simulink model "Inverter_Bipolar_motor"  (R2024a)
settings: Solver=VariableStepAuto  StartTime=0.0  StopTime=2  RelTol=1e-3
undefined symbols (not defined in the file): Capacitor, Start
libraries: spsIGBTDiodeLib x4, spsCurrentMeasurementLib x2, spsDCVoltageSourceLib x1, simulink x1, spsSinglePhaseAsynchronousMachineLib x1, spsVoltageMeasurementLib x1, sps_lib x1
settings Model: Creator=yashg  LastModifiedBy=yashg

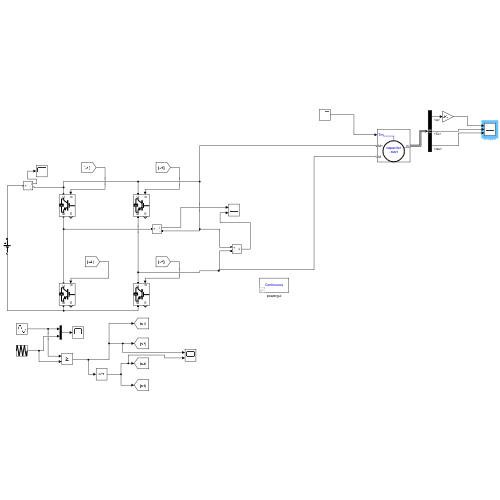
[thumbnail: Simulink's stored preview of the top-level diagram]
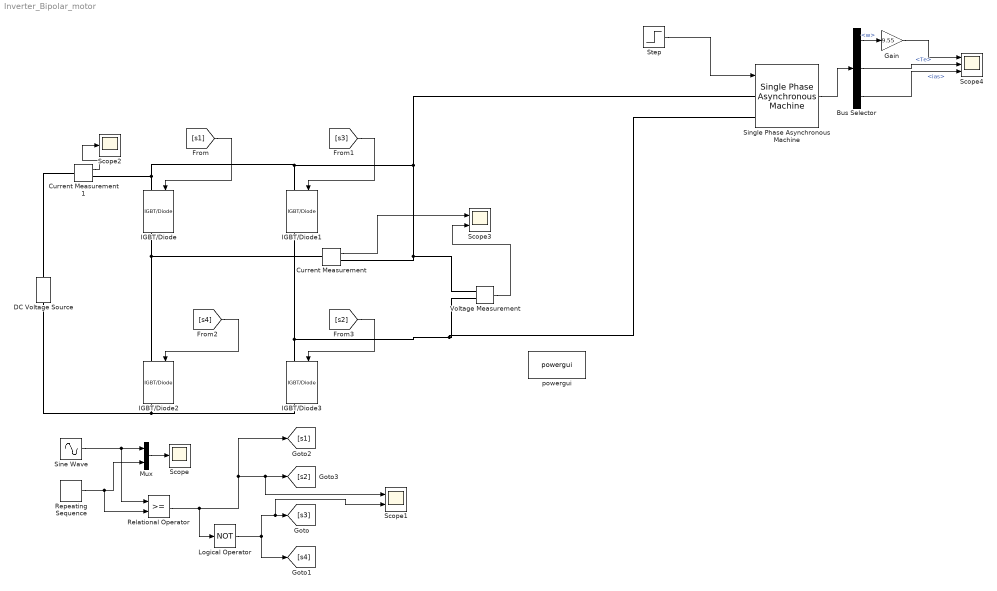
== system Inverter_Bipolar_motor ==
  Bus Selector : BusSelector  OutputSignals=w,Te,ias
  Current Measurement : spsCurrentMeasurementLib/Current Measurement  PhasorSimulation=off  OutputType=Complex  PSBequivalent=0
  Current Measurement1 : spsCurrentMeasurementLib/Current Measurement  PhasorSimulation=off  OutputType=Complex  PSBequivalent=0
  DC Voltage Source : spsDCVoltageSourceLib/DC Voltage Source  Amplitude=100  Measurements=None
  Gain : Gain  Gain=9.55
  IGBT/Diode{,1..3} (4 alike) : spsIGBTDiodeLib/IGBT//Diode  Ron=1e-3  Rs=1e5  Cs=inf  Measurements=on
  Logical Operator : Logic  Operator=NOT  AllPortsSameDT=off  OutDataTypeStr=boolean
  Mux : Mux  Inputs=2
  Relational Operator : RelationalOperator  OutDataTypeStr=boolean  RndMeth=Simplest  InputSameDT=off
  Repeating Sequence : simulink/Sources/Repeating Sequence  rep_seq_t=[0 1 2 3 4]*[1/400]  rep_seq_y=[0 1 0 -1 0]
  Scope : Scope
  Scope1 : Scope  NumInputPorts=2
  Scope2 : Scope
  Scope3 : Scope  NumInputPorts=2
  Scope4 : Scope  NumInputPorts=3
  Sine Wave : Sin  Frequency=2*pi*50  SampleTime=0
  Single Phase Asynchronous Machine : spsSinglePhaseAsynchronousMachineLib/Single Phase Asynchronous Machine  MechanicalLoad=Torque Tm  UNITS=SI  MachineType=Capacitor-Start  MeasurementBus=on  NominalParameters="[ .25*746  110  60]"  MainWindingStator="[2.02  7.4e-3]"  MainWindingRotor="[4.12  5.6e-3]"  MutualInductance=0.1772  AuxiliaryWinding="[7.14  8.5e-3]"  Mechanical="[0.0146  0  2 1.18]"  CapacitorStart="[2  254.7e-6]"  CapacitorRun="[18  21.1e-6]"  DisconnectionSpeed=75  InitialSpeed=0  DataType=SI  TsPowergui=0  TsBlock=-1
      settings: LibrarySourceBlock=|
      | sps_lib/Electrical Machines/Single Phase
      | Asynchronous Machine
  Step : Step  Time=0  After=10  SampleTime=0
  Voltage Measurement : spsVoltageMeasurementLib/Voltage Measurement  PhasorSimulation=off  OutputType=Complex  PSBequivalent=0
  powergui : sps_lib/powergui  Priority=1  SimulationMode=Continuous  SampleTime=50e-6  frequency=60  Iterations=50  frequencyindice=0  Pbase=100e6  ErrMax=1e-4  UnitsV=kV  UnitsW=MW  buscounter=0  FunctionMessages=off  echomessages=off  EnableUseOfTLC=off  CurrentSourceSwitches=off  DisableSnubberDevices=off  DisableRonSwitches=off  DisableVfSwitches=off  DisplayEquations=off  AutomaticDiscreteSolvers=off  SolverType=Tustin/Backward Euler (TBE)  Interpol=off  ExternalGateDelay=off  methode=off  Ts=100  x0status=blocks  SPID=on  SwTol=0  HookPort=off  NonlinearTolerance=1e-4  nMaxIteration=100  ContinueOnMaxIteration=off  RestoreLinks=warning  ResistiveCurrentMeasurement=off  Frange=[0:2:500]  Ylog=off  Xlog=on  ShowGrid=off  save=off  variable=ZData  structure=0  ZoomFFT=off  StartTime=0.0  cycles=1  DisplayStyle=1  fundamental=60  FreqAxis=off  MaxFrequency=1000  frequencyindicesteady=1  RmsSteady=1  display=off
  wires:
  Mux/1 -> Scope/1
  Relational Operator/1 -> Logical Operator/1, Scope1/1, [s2], [s1]
  [s4] -> IGBT/Diode2/1
  [s3] -> IGBT/Diode1/1
  Current Measurement/1 -> Scope3/1
  Voltage Measurement/1 -> Scope3/2
  [s1] -> IGBT/Diode/1
  [s2] -> IGBT/Diode3/1
  Repeating Sequence/1 -> Relational Operator/2, Mux/2
  Logical Operator/1 -> [s4], Scope1/2, [s3]
  Current Measurement1/1 -> Scope2/1
  Sine Wave/1 -> Relational Operator/1, Mux/1
  Step/1 -> Single Phase Asynchronous Machine/1
  Bus Selector/2 -> Scope4/2  "<Te>"
  Gain/1 -> Scope4/1
  Bus Selector/1 -> Gain/1  "<w>"
  Bus Selector/3 -> Scope4/3  "<ias>"
  Single Phase Asynchronous Machine/1 -> Bus Selector/1
  connections:
  IGBT/Diode2/LConn1 -- IGBT/Diode/RConn1 -- Current Measurement/LConn1
  DC Voltage Source/LConn1 -- IGBT/Diode2/RConn1 -- IGBT/Diode3/RConn1
  Current Measurement/RConn1 -- Single Phase Asynchronous Machine/LConn1 -- Current Measurement1/RConn1 -- IGBT/Diode/LConn1 -- IGBT/Diode1/LConn1 -- Voltage Measurement/LConn1
  IGBT/Diode3/LConn1 -- Single Phase Asynchronous Machine/LConn2 -- Voltage Measurement/LConn2 -- IGBT/Diode1/RConn1
  DC Voltage Source/RConn1 -- Current Measurement1/LConn1
